simulink model "jointSpaceGravityCompensation"  (R2020b)
settings: Solver=VariableStepAuto  StartTime=0.0  StopTime=3  RelTol=1e-3
values from neighbouring files (symbols this model uses):
  KD = diag([ 20  10  21])    [parameters.m]
  KP = diag([240 240 200])    [parameters.m]
libraries: vrlib x1
settings Model: Creator=Edoardo  LastModifiedBy=Edoardo

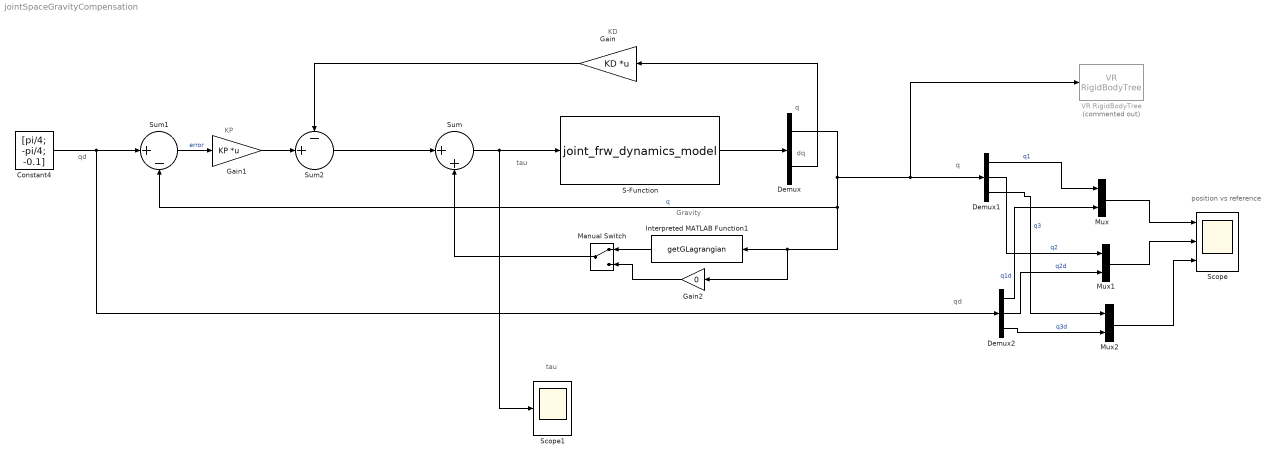
== system jointSpaceGravityCompensation ==
  note: tau
  note: Gravity
  note: position vs reference
  note: q
  note: qd
  note: tau
  note: KP
  note: KD
  note: qd
  note: dq
  note: q
  Constant4 : Constant  Value=[pi/4; -pi/4; -0.1]  VectorParams1D=off
  Demux : Demux  Outputs=2
  Demux1 : Demux  Outputs=3
  Demux2 : Demux  Outputs=3
  Gain : Gain  Gain=KD  Multiplication=Matrix(K*u) (u vector)
  Gain1 : Gain  Gain=KP  Multiplication=Matrix(K*u) (u vector)
  Gain2 : Gain  Gain=0
  Interpreted MATLAB Function1 : MATLABFcn  MATLABFcn=getGLagrangian
  Manual Switch : ManualSwitch
  Mux : Mux  Inputs=2
  Mux1 : Mux  Inputs=2
  Mux2 : Mux  Inputs=2
  S-Function : S-Function  FunctionName=joint_frw_dynamics_model  Parameters=myRobot  SFunctionDeploymentMode=off  EnableBusSupport=off
  Scope : Scope  NumInputPorts=3
  Scope1 : Scope
  Sum : Sum  Inputs=|++
  Sum1 : Sum  Inputs=|+-
  Sum2 : Sum  Inputs=-+|
  VR RigidBodyTree : vrlib/VR RigidBodyTree  Commented=on  RBT=robot  useRBT=on  Ts=-1  ForceViewerOpen=on
      settings: SourceProductBaseCode=SL
  wires:
  S-Function/1 -> Demux/1
  Sum/1 -> Scope1/1, S-Function/1
  Demux/2 -> Gain/1
  Sum2/1 -> Sum/1
  Gain/1 -> Sum2/1
  Sum1/1 -> Gain1/1  "error"
  Demux/1 -> Interpreted MATLAB Function1/1, Gain2/1, Sum1/2, Demux1/1, VR RigidBodyTree/1  "q"
  Gain1/1 -> Sum2/2
  Constant4/1 -> Demux2/1, Sum1/1
  Demux1/1 -> Mux/1  "q1"
  Demux1/3 -> Mux2/1  "q3"
  Demux2/1 -> Mux/2  "q1d"
  Demux2/2 -> Mux1/2  "q2d"
  Demux2/3 -> Mux2/2  "q3d"
  Mux/1 -> Scope/1
  Mux1/1 -> Scope/2
  Mux2/1 -> Scope/3
  Demux1/2 -> Mux1/1  "q2"
  Gain2/1 -> Manual Switch/2
  Manual Switch/1 -> Sum/2
  Interpreted MATLAB Function1/1 -> Manual Switch/1
